simulink model "TST_SpdDemSwt_VD"  (R2016b)
settings: Solver=FixedStepDiscrete  StartTime=0.0  StopTime=simTime  FixedStep=sampleTime  RelTol=1e-3
values from neighbouring files (symbols this model uses):
  testCase = 1    [initTST_SpdDemSwt_VD_001.m]    (also in initTST_SpdDemSwt_VD_002.m = 2)
libraries: simulink x5, UnitTest_Lib x2
settings Model: Creator=zhengjinyan  LastModifiedBy=zhengjinyan
settings DebuggingCC: SignalRangeChecking=error

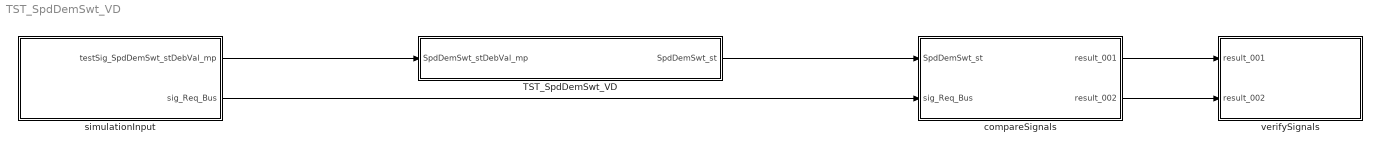
== system TST_SpdDemSwt_VD ==
  TST_SpdDemSwt_VD : Subsystem
  compareSignals : Subsystem
  simulationInput : Subsystem
  verifySignals : Subsystem
  wires:
  simulationInput/1(testSig_SpdDemSwt_stDebVal_mp) -> TST_SpdDemSwt_VD/1(SpdDemSwt_stDebVal_mp)
  TST_SpdDemSwt_VD/1(SpdDemSwt_st) -> compareSignals/1(SpdDemSwt_st)
  simulationInput/2(sig_Req_Bus) -> compareSignals/2(sig_Req_Bus)
  compareSignals/1(result_001) -> verifySignals/1(result_001)
  compareSignals/2(result_002) -> verifySignals/2(result_002)

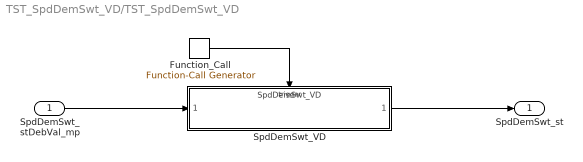
== system TST_SpdDemSwt_VD/TST_SpdDemSwt_VD ==
  SpdDemSwt_stDebVal_mp : Inport
  Function_Call : simulink/Ports & Subsystems/Function-Call Generator  sample_time=sampleTime  numberOfIterations=1
  SpdDemSwt_VD : ModelReference  ModelNameDialog=SpdDemSwt_VD  SimulationMode=Normal  ModelReferenceVersion=1.3  TriggerPortName=function  TriggerPortTriggerType=function-call  TriggerPortStatesWhenEnabling=held
  SpdDemSwt_st : Outport
  wires:
  Function_Call/1 -> SpdDemSwt_VD/Trigger
  SpdDemSwt_stDebVal_mp/1 -> SpdDemSwt_VD/1
  SpdDemSwt_VD/1 -> SpdDemSwt_st/1

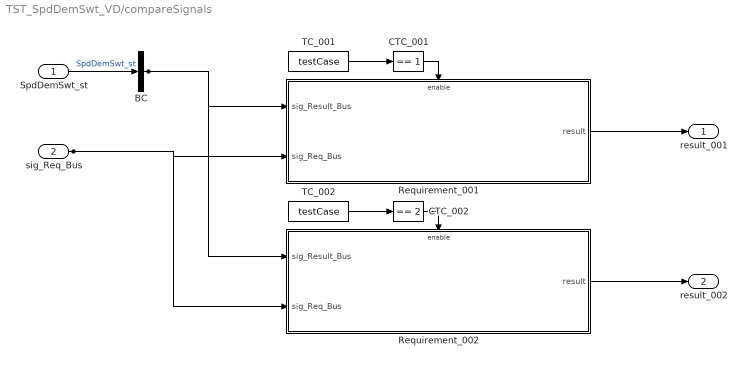
== system TST_SpdDemSwt_VD/compareSignals ==
  SpdDemSwt_st : Inport
  sig_Req_Bus : Inport  Port=2
  BC : BusCreator  Inputs=1
  CTC_001 : simulink/Logic and Bit Operations/Compare To Constant  relop===  const=1  OutDataTypeStr=boolean
  CTC_002 : simulink/Logic and Bit Operations/Compare To Constant  relop===  const=2  OutDataTypeStr=boolean
  Requirement_001 : Subsystem
  Requirement_002 : Subsystem
  TC_001 : Constant  Value=testCase
  TC_002 : Constant  Value=testCase
  result_001 : Outport
  result_002 : Outport  Port=2
  wires:
  SpdDemSwt_st/1 -> BC/1  "SpdDemSwt_st"
  TC_001/1 -> CTC_001/1
  CTC_001/1 -> Requirement_001/Enable
  sig_Req_Bus/1 -> Requirement_001/2(sig_Req_Bus), Requirement_002/2(sig_Req_Bus)
  BC/1 -> Requirement_001/1(sig_Result_Bus), Requirement_002/1(sig_Result_Bus)
  Requirement_001/1(result) -> result_001/1
  TC_002/1 -> CTC_002/1
  CTC_002/1 -> Requirement_002/Enable
  Requirement_002/1(result) -> result_002/1

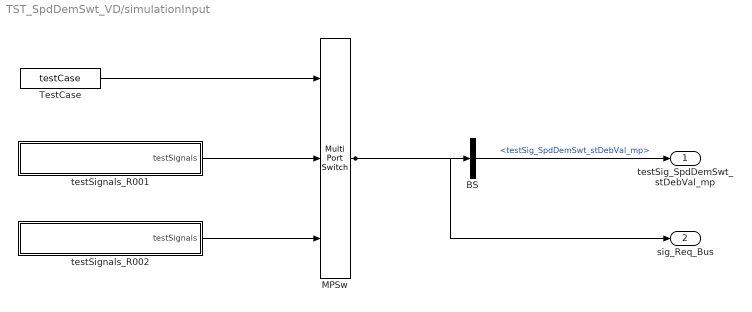
== system TST_SpdDemSwt_VD/simulationInput ==
  BS : BusSelector  OutputSignals=testSig_SpdDemSwt_stDebVal_mp
  MPSw : MultiPortSwitch  Inputs=2  SaturateOnIntegerOverflow=on  InputSameDT=on
  TestCase : Constant  Value=testCase
  testSignals_R001 : Subsystem
  testSignals_R002 : Subsystem
  testSig_SpdDemSwt_stDebVal_mp : Outport
  sig_Req_Bus : Outport  Port=2
  wires:
  BS/1 -> testSig_SpdDemSwt_stDebVal_mp/1  "<testSig_SpdDemSwt_stDebVal_mp>"
  MPSw/1 -> BS/1, sig_Req_Bus/1
  TestCase/1 -> MPSw/1
  testSignals_R001/1(testSignals) -> MPSw/2
  testSignals_R002/1(testSignals) -> MPSw/3

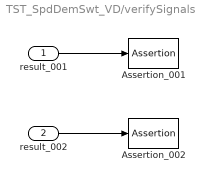
== system TST_SpdDemSwt_VD/verifySignals ==
  result_001 : Inport
  result_002 : Inport  Port=2
  Assertion_001 : Assertion  Enabled=off
  Assertion_002 : Assertion  Enabled=off
  wires:
  result_001/1 -> Assertion_001/1
  result_002/1 -> Assertion_002/1

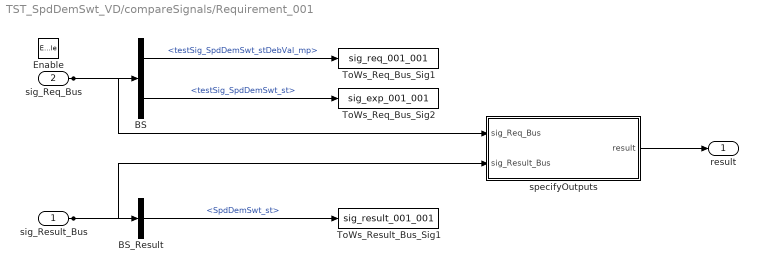
== system TST_SpdDemSwt_VD/compareSignals/Requirement_001 ==
  sig_Result_Bus : Inport
  sig_Req_Bus : Inport  Port=2
  Enable : EnablePort
  BS : BusSelector  OutputSignals=testSig_SpdDemSwt_stDebVal_mp,testSig_SpdDemSwt_st
  BS_Result : BusSelector  OutputSignals=SpdDemSwt_st
  ToWs_Req_Bus_Sig1 : ToWorkspace  VariableName=sig_req_001_001  SaveFormat=Structure With Time
  ToWs_Req_Bus_Sig2 : ToWorkspace  VariableName=sig_exp_001_001  SaveFormat=Structure With Time
  ToWs_Result_Bus_Sig1 : ToWorkspace  VariableName=sig_result_001_001  SaveFormat=Structure With Time
  specifyOutputs : Subsystem
  result : Outport
  wires:
  sig_Req_Bus/1 -> BS/1, specifyOutputs/1(sig_Req_Bus)
  BS/1 -> ToWs_Req_Bus_Sig1/1  "<testSig_SpdDemSwt_stDebVal_mp>"
  BS/2 -> ToWs_Req_Bus_Sig2/1  "<testSig_SpdDemSwt_st>"
  sig_Result_Bus/1 -> BS_Result/1, specifyOutputs/2(sig_Result_Bus)
  BS_Result/1 -> ToWs_Result_Bus_Sig1/1  "<SpdDemSwt_st>"
  specifyOutputs/1(result) -> result/1

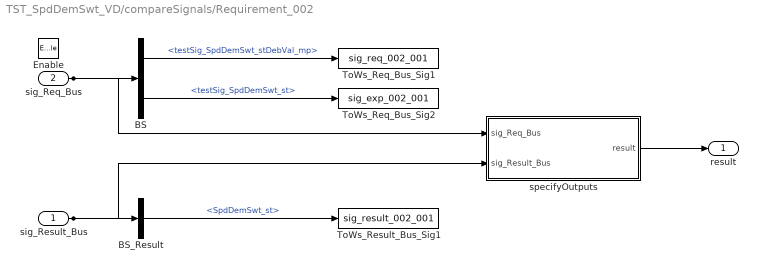
== system TST_SpdDemSwt_VD/compareSignals/Requirement_002 ==
  sig_Result_Bus : Inport
  sig_Req_Bus : Inport  Port=2
  Enable : EnablePort
  BS : BusSelector  OutputSignals=testSig_SpdDemSwt_stDebVal_mp,testSig_SpdDemSwt_st
  BS_Result : BusSelector  OutputSignals=SpdDemSwt_st
  ToWs_Req_Bus_Sig1 : ToWorkspace  VariableName=sig_req_002_001  SaveFormat=Structure With Time
  ToWs_Req_Bus_Sig2 : ToWorkspace  VariableName=sig_exp_002_001  SaveFormat=Structure With Time
  ToWs_Result_Bus_Sig1 : ToWorkspace  VariableName=sig_result_002_001  SaveFormat=Structure With Time
  specifyOutputs : Subsystem
  result : Outport
  wires:
  sig_Req_Bus/1 -> BS/1, specifyOutputs/1(sig_Req_Bus)
  BS/1 -> ToWs_Req_Bus_Sig1/1  "<testSig_SpdDemSwt_stDebVal_mp>"
  BS/2 -> ToWs_Req_Bus_Sig2/1  "<testSig_SpdDemSwt_st>"
  sig_Result_Bus/1 -> BS_Result/1, specifyOutputs/2(sig_Result_Bus)
  BS_Result/1 -> ToWs_Result_Bus_Sig1/1  "<SpdDemSwt_st>"
  specifyOutputs/1(result) -> result/1

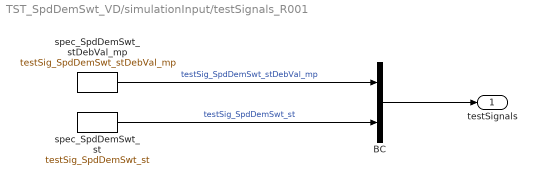
== system TST_SpdDemSwt_VD/simulationInput/testSignals_R001 ==
  BC : BusCreator  Inputs=2
  spec_SpdDemSwt_st : FromWorkspace  VariableName=testSig_SpdDemSwt_st  Interpolate=off  OutputAfterFinalValue=Holding final value
  spec_SpdDemSwt_stDebVal_mp : FromWorkspace  VariableName=testSig_SpdDemSwt_stDebVal_mp  Interpolate=off  OutputAfterFinalValue=Holding final value
  testSignals : Outport
  wires:
  BC/1 -> testSignals/1
  spec_SpdDemSwt_stDebVal_mp/1 -> BC/1  "testSig_SpdDemSwt_stDebVal_mp"
  spec_SpdDemSwt_st/1 -> BC/2  "testSig_SpdDemSwt_st"

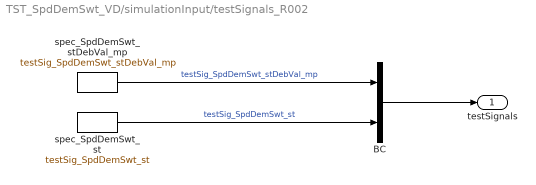
== system TST_SpdDemSwt_VD/simulationInput/testSignals_R002 ==
  BC : BusCreator  Inputs=2
  spec_SpdDemSwt_st : FromWorkspace  VariableName=testSig_SpdDemSwt_st  Interpolate=off  OutputAfterFinalValue=Holding final value
  spec_SpdDemSwt_stDebVal_mp : FromWorkspace  VariableName=testSig_SpdDemSwt_stDebVal_mp  Interpolate=off  OutputAfterFinalValue=Holding final value
  testSignals : Outport
  wires:
  BC/1 -> testSignals/1
  spec_SpdDemSwt_stDebVal_mp/1 -> BC/1  "testSig_SpdDemSwt_stDebVal_mp"
  spec_SpdDemSwt_st/1 -> BC/2  "testSig_SpdDemSwt_st"

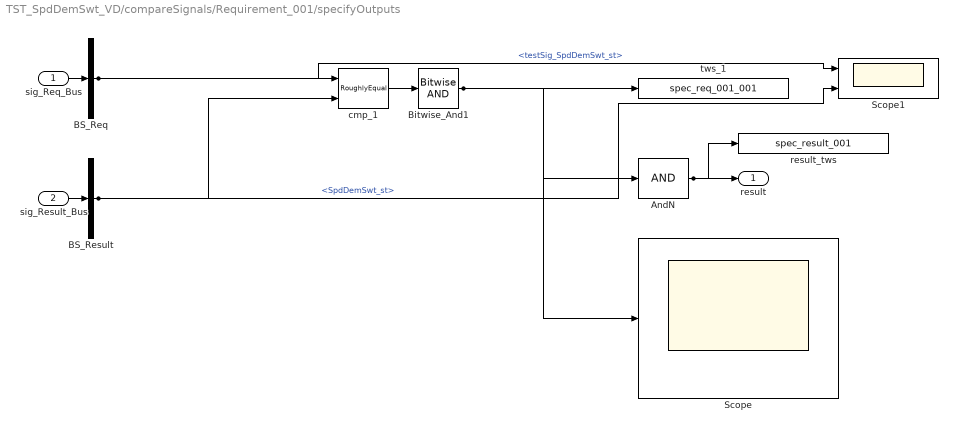
== system TST_SpdDemSwt_VD/compareSignals/Requirement_001/specifyOutputs ==
  sig_Req_Bus : Inport
  sig_Result_Bus : Inport  Port=2
  AndN : Logic  Inputs=1
  BS_Req : BusSelector  OutputSignals=testSig_SpdDemSwt_st
  BS_Result : BusSelector  OutputSignals=SpdDemSwt_st
  Bitwise_And1 : simulink/Logic and Bit Operations/Bitwise Operator  logicop=AND  UseBitMask=off  BitMask=bin2dec('11011001')  BitMaskRealWorld=Stored Integer
  Scope : Scope
  Scope1 : Scope  NumInputPorts=2
  cmp_1 : UnitTest_Lib/RoughlyEqual  slope=0.1
  result_tws : ToWorkspace  VariableName=spec_result_001
  tws_1 : ToWorkspace  VariableName=spec_req_001_001
  result : Outport
  wires:
  sig_Req_Bus/1 -> BS_Req/1
  sig_Result_Bus/1 -> BS_Result/1
  AndN/1 -> result/1, result_tws/1
  BS_Req/1 -> cmp_1/1, Scope1/1  "<testSig_SpdDemSwt_st>"
  BS_Result/1 -> cmp_1/2, Scope1/2  "<SpdDemSwt_st>"
  cmp_1/1 -> Bitwise_And1/1
  Bitwise_And1/1 -> tws_1/1, AndN/1, Scope/1

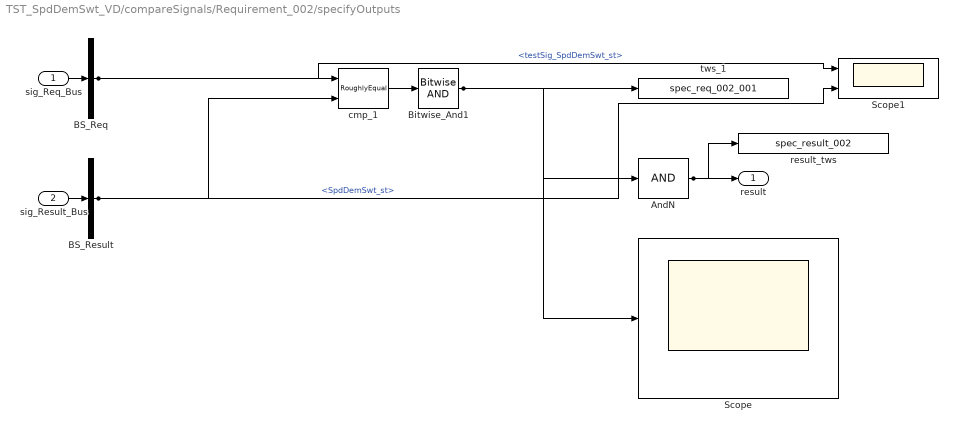
== system TST_SpdDemSwt_VD/compareSignals/Requirement_002/specifyOutputs ==
  sig_Req_Bus : Inport
  sig_Result_Bus : Inport  Port=2
  AndN : Logic  Inputs=1
  BS_Req : BusSelector  OutputSignals=testSig_SpdDemSwt_st
  BS_Result : BusSelector  OutputSignals=SpdDemSwt_st
  Bitwise_And1 : simulink/Logic and Bit Operations/Bitwise Operator  logicop=AND  UseBitMask=off  BitMask=bin2dec('11011001')  BitMaskRealWorld=Stored Integer
  Scope : Scope
  Scope1 : Scope  NumInputPorts=2
  cmp_1 : UnitTest_Lib/RoughlyEqual  slope=0.1
  result_tws : ToWorkspace  VariableName=spec_result_002
  tws_1 : ToWorkspace  VariableName=spec_req_002_001
  result : Outport
  wires:
  sig_Req_Bus/1 -> BS_Req/1
  sig_Result_Bus/1 -> BS_Result/1
  AndN/1 -> result/1, result_tws/1
  BS_Req/1 -> cmp_1/1, Scope1/1  "<testSig_SpdDemSwt_st>"
  BS_Result/1 -> cmp_1/2, Scope1/2  "<SpdDemSwt_st>"
  cmp_1/1 -> Bitwise_And1/1
  Bitwise_And1/1 -> tws_1/1, AndN/1, Scope/1
